simulink model "stand_nove"  (R2021a)
settings: Solver=VariableStepAuto  StartTime=0.0  StopTime=3.0  RelTol=1e-3
values from neighbouring files (symbols this model uses):
  fn = 50    [stand_final.m]
  Jm = 0.0019    [stand_final.m]
  pp = 2    [stand_final.m]
  Un = 23.4    [stand_final.m]
  X0 = 0    [stand_final.m]
libraries: General x38, nesl_utility x16, Math x12, ee_lib x11, fl_lib x11, Control x4, MotorControl x3, Basic x1
settings Model: Creator=pavel  LastModifiedBy=pavel

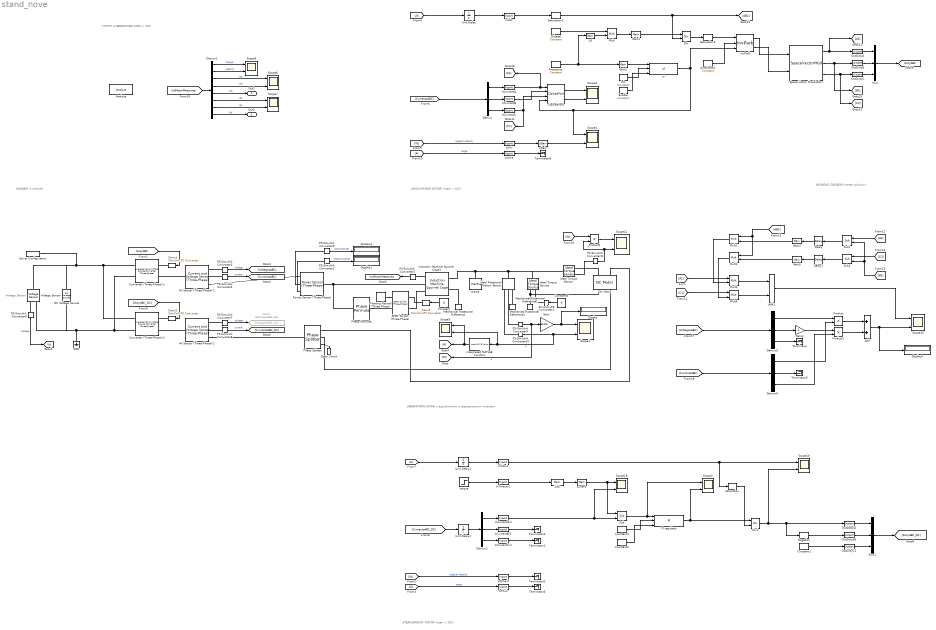
== system stand_nove ==
  note: ASYNCHRONNI MOTOR
      | (rizeni v X2C)
  note: LABORATORNI STAND
      | s asynchronnim a stejnosmernym motorem
  note: Voltage Sensor
  note: STEJNOSMERNY MOTOR
      | (rizeni v X2C)
  note: NAPAJENI
      | (z menice)
  note: ARONOVO ZAPOJENI
      | (mereni prikonu)
  note: VYSTUP a GENEROVANI KODU v X2C
  1/cfi : General/Gain  Gain=1/0.06  M2CAutoParam_UsedImplementation=32 Bit Floating Point  x2c_cfg_enableStaticId=off  x2c_cfg_staticId=1  x2c_cfg_enableCot=off  BlockName=Gain
      settings: SourceProductName=X2C General
  1/f : General/Gain  Gain=1/fn  M2CAutoParam_UsedImplementation=32 Bit Floating Point  x2c_cfg_enableStaticId=off  x2c_cfg_staticId=1  x2c_cfg_enableCot=off  BlockName=Gain
      settings: SourceProductName=X2C General
  AV Sensor (Three-Phase)-1 : ee_lib/Sensors & Transducers/Current and Voltage Sensor (Three-Phase)  vMeasurementType=ee.enum.vmeasurement.ll  outputUnit=ee.enum.unit.si  SRated=100e6 V*A  VRated=24e3 V  I_specify=off  I_priority=None  I=[ 0 0 0 ] A  I_nominal_specify=off  I_nominal_unit=A  I_nominal_value=1  V_specify=off  V_priority=None  V=[ 0 0 0 ] V  V_nominal_specify=off  V_nominal_unit=V  V_nominal_value=1
      settings: SourceProductBaseCode=PS  InternalSimscapePortConfiguration="{\"Bottom\":[],\"Left\":[{\"id\":\"N1\",\"label\":\"~1\",\"type\":\"foundation.electrical.three_phase\"}],\"Right\":[{\"id\":\"V_output\",\"label\":\"V\",\"type\":\"output\"},{\"id\":\"I_output\",\"label\":\"I\",\"type\":\"output\"},{\"id\":\"N2\",\"label\":\"~2\",\"type\":\"foundation.electrical.three_phase\"}],\"Top\":[]}"
  AV Sensor (Three-Phase)-2 : ee_lib/Sensors & Transducers/Current and Voltage Sensor (Three-Phase)  vMeasurementType=ee.enum.vmeasurement.ll  outputUnit=ee.enum.unit.si  SRated=100e6 V*A  VRated=24e3 V  I_specify=off  I_priority=None  I=[ 0 0 0 ] A  I_nominal_specify=off  I_nominal_unit=A  I_nominal_value=1  V_specify=off  V_priority=None  V=[ 0 0 0 ] V  V_nominal_specify=off  V_nominal_unit=V  V_nominal_value=1
      settings: SourceProductBaseCode=PS  InternalSimscapePortConfiguration="{\"Bottom\":[],\"Left\":[{\"id\":\"N1\",\"label\":\"~1\",\"type\":\"foundation.electrical.three_phase\"}],\"Right\":[{\"id\":\"V_output\",\"label\":\"V\",\"type\":\"output\"},{\"id\":\"I_output\",\"label\":\"I\",\"type\":\"output\"},{\"id\":\"N2\",\"label\":\"~2\",\"type\":\"foundation.electrical.three_phase\"}],\"Top\":[]}"
  Add : Sum
  Add1 : Math/Add  M2CAutoParam_UsedImplementation=32 Bit Floating Point  x2c_cfg_enableStaticId=off  x2c_cfg_staticId=1  x2c_cfg_enableCot=off  BlockName=Add
      settings: SourceProductName=X2C Math
  Amplitude1 : General/Constant  Value=0  M2CAutoParam_UsedImplementation=32 Bit Floating Point  x2c_cfg_enableStaticId=off  x2c_cfg_staticId=1  x2c_cfg_enableCot=off  BlockName=Constant
      settings: SourceProductName=X2C General
  Analyze : Basic/Analyze
      settings: SourceProductName=X2C Basic
  ClarkeNPark : MotorControl/ClarkeNPark  M2CAutoParam_UsedImplementation=32 Bit Floating Point  x2c_cfg_enableStaticId=off  x2c_cfg_staticId=1  x2c_cfg_enableCot=off  BlockName=ClarkeNPark
      settings: SourceProductName=X2C MotorControl
  Constant : Constant  Value=0
  Constant1 : General/Constant  Value=0.0  M2CAutoParam_UsedImplementation=32 Bit Floating Point  x2c_cfg_enableStaticId=off  x2c_cfg_staticId=1  x2c_cfg_enableCot=off  BlockName=Constant
      settings: SourceProductName=X2C General
  Constant3 : General/Constant  Value=1  M2CAutoParam_UsedImplementation=Boolean  x2c_cfg_enableStaticId=off  x2c_cfg_staticId=1  x2c_cfg_enableCot=off  BlockName=Constant
      settings: SourceProductName=X2C General
  Constant4 : General/Constant  Value=0.0  M2CAutoParam_UsedImplementation=32 Bit Floating Point  x2c_cfg_enableStaticId=off  x2c_cfg_staticId=1  x2c_cfg_enableCot=off  BlockName=Constant
      settings: SourceProductName=X2C General
  Constant6 : Constant  Value=0
  Conv1 : nesl_utility/Simulink-PS Converter  PhysicalDomain=network_engine_domain  SubClassName=ps_input  LeftPortType=input  RightPortType=output  PseudoPeriodic=off  Frequencies=[]  NoiseDistribution=none  NoiseParameters=[]  Unit=1  AffineConversion=off  FilteringAndDerivatives=provide  SimscapeFilterOrder=1  InputFilterTimeConstant=0.001  UdotUserProvided=0
      settings: SourceProductBaseCode=PW,SS
  Conv2 : nesl_utility/Simulink-PS Converter  PhysicalDomain=network_engine_domain  SubClassName=ps_input  LeftPortType=input  RightPortType=output  PseudoPeriodic=off  Frequencies=[]  NoiseDistribution=none  NoiseParameters=[]  Unit=1  AffineConversion=off  FilteringAndDerivatives=provide  SimscapeFilterOrder=1  InputFilterTimeConstant=0.001  UdotUserProvided=0
      settings: SourceProductBaseCode=PW,SS
  Conv3 : nesl_utility/Simulink-PS Converter  PhysicalDomain=network_engine_domain  SubClassName=ps_input  LeftPortType=input  RightPortType=output  PseudoPeriodic=off  Frequencies=[]  NoiseDistribution=none  NoiseParameters=[]  Unit=1  AffineConversion=off  FilteringAndDerivatives=provide  SimscapeFilterOrder=1  InputFilterTimeConstant=0.001  UdotUserProvided=0
      settings: SourceProductBaseCode=PW,SS
  Converter (Three-Phase)-1 : ee_lib/Semiconductors & Converters/Converters/Average-Value Voltage Source Converter (Three-Phase)  losses_parameterization=ee.enum.converters.losses.fixed  Pfixed=0.0001 W  ks=0.01  kc1=1.7 V  kc2=0.01 Ohm  Ploss_vect=[100, 800, 1870, 3250, 4900] W  Irms_vect=[10, 100, 200, 300, 400] A  Vdc_nom=300 V  thermal_mass=30000 J/K  temperature_specify=off  temperature_priority=High  temperature=298.15 K  temperature_nominal_specify=off  temperature_nominal_unit=K  temperature_nominal_value=1
      settings: SourceProductBaseCode=PS  InternalSimscapePortConfiguration="{\"Bottom\":[],\"Left\":[{\"id\":\"ModWave\",\"label\":\"ModWave\",\"type\":\"input\"},{\"id\":\"N\",\"label\":\"~\",\"type\":\"foundation.electrical.three_phase\"}],\"Right\":[{\"id\":\"p\",\"label\":\"+\",\"type\":\"foundation.electrical.electrical\"},{\"id\":\"n\",\"label\":\"-\",\"type\":\"foundation.electrical.electrical\"}],\"Top\":[]}"
  Converter (Three-Phase)-2 : ee_lib/Semiconductors & Converters/Converters/Average-Value Voltage Source Converter (Three-Phase)  losses_parameterization=ee.enum.converters.losses.fixed  Pfixed=0.1 W  ks=0.01  kc1=1.7 V  kc2=0.01 Ohm  Ploss_vect=[100, 800, 1870, 3250, 4900] W  Irms_vect=[10, 100, 200, 300, 400] A  Vdc_nom=300 V  thermal_mass=30000 J/K  temperature_specify=off  temperature_priority=High  temperature=298.15 K  temperature_nominal_specify=off  temperature_nominal_unit=K  temperature_nominal_value=1
      settings: SourceProductBaseCode=PS  InternalSimscapePortConfiguration="{\"Bottom\":[],\"Left\":[{\"id\":\"ModWave\",\"label\":\"ModWave\",\"type\":\"input\"},{\"id\":\"N\",\"label\":\"~\",\"type\":\"foundation.electrical.three_phase\"}],\"Right\":[{\"id\":\"p\",\"label\":\"+\",\"type\":\"foundation.electrical.electrical\"},{\"id\":\"n\",\"label\":\"-\",\"type\":\"foundation.electrical.electrical\"}],\"Top\":[]}"
  DC Voltage Source : fl_lib/Electrical/Electrical Sources/DC Voltage Source  v0=Ud V
  DC Motor : ee_lib/Electromechanical/Brushed Motors/DC Motor  field_option=ee.enum.field_option.pm  Rf=100 Ohm  Lf=1 H  Laf=0.15 H  If0=0 A  parameterization=ee.enum.dcparam_option.circuit_param  Ra=Ra Ohm  La=La H  emf_or_torque=ee.enum.emf_or_torque.kv  Kv=cfi V/(rad/s)  Ki=6.876e-4 N*m/A  T_stall=0.24e-3 N*m  w_max=19100 rpm  w_rated=15000 rpm  P_rated=0.08 W  V_rated=1.5 V  J=Jm kg*m^2  lam_param=ee.enum.lam_param.damping  lam=0 N*m/(rad/s)  i_noload=0 A  V_i_noload=1.5 V  speed0=0 rpm  enable_fault_armature=ee.enum.faults.faultEnable.no  rev_faulted=1 / 3  G_faulted_armature=1e-5 S  fault_trigger_armature=ee.enum.faults.faultTrigger.temporal  t_fault_armature=1 s  max_permissible_current_armature=inf A  t_fail_on_current_armature=1 s  enable_fault_field=ee.enum.faults.faultEnable.no  G_faulted_field=1e-5 S  fault_trigger_field=ee.enum.faults.faultTrigger.temporal  t_fault_field=1 s  max_permissible_current_field=inf A  t_fail_on_current_field=1 s  fault_action=ee.enum.faults.faultAction.none  alpha=3.93e-3 1/K  Tmeas=25 degC  thermal_mass=100 J/K  initial_temperature=25 degC
  Delay : Control/Delay  ts_fact=1.0  M2CAutoParam_UsedImplementation=32 Bit Floating Point  x2c_cfg_enableStaticId=off  x2c_cfg_staticId=1  x2c_cfg_enableCot=off  BlockName=Delay
      settings: SourceProductName=X2C Control
  Delay1 : Control/Delay  ts_fact=1.0  M2CAutoParam_UsedImplementation=32 Bit Floating Point  x2c_cfg_enableStaticId=off  x2c_cfg_staticId=1  x2c_cfg_enableCot=off  BlockName=Delay
      settings: SourceProductName=X2C Control
  Demux{,2,5..6} (4 alike) : Demux  Outputs=3
  Demux1 : Demux  Outputs=8
  Display{,1,3..4} (4 alike) : Display
  Div : Math/Div  M2CAutoParam_UsedImplementation=32 Bit Floating Point  x2c_cfg_enableStaticId=off  x2c_cfg_staticId=1  x2c_cfg_enableCot=off  BlockName=Div
      settings: SourceProductName=X2C Math
  Div1 : Math/Div  M2CAutoParam_UsedImplementation=32 Bit Floating Point  x2c_cfg_enableStaticId=off  x2c_cfg_staticId=1  x2c_cfg_enableCot=off  BlockName=Div
      settings: SourceProductName=X2C Math
  Enable : General/Constant  Value=1  M2CAutoParam_UsedImplementation=Boolean  x2c_cfg_enableStaticId=off  x2c_cfg_staticId=1  x2c_cfg_enableCot=off  BlockName=Constant
      settings: SourceProductName=X2C General
  Floating Neutral (Three-Phase) : ee_lib/Connectors & References/Floating Neutral (Three-Phase)  G_parasitic=1e-12 1/Ohm
      settings: SourceProductBaseCode=PS  InternalSimscapePortConfiguration="{\"Bottom\":[],\"Left\":[{\"id\":\"N\",\"label\":\"~\",\"type\":\"foundation.electrical.three_phase\"}],\"Right\":[],\"Top\":[]}"
  Frequency : General/Constant  Value=fn  M2CAutoParam_UsedImplementation=32 Bit Floating Point  x2c_cfg_enableStaticId=off  x2c_cfg_staticId=1  x2c_cfg_enableCot=off  BlockName=Constant
      settings: SourceProductName=X2C General
  GND : fl_lib/Electrical/Electrical Elements/Electrical Reference
  Gain : Gain  Gain=60/2/pi
  Gain1 : General/Gain  Gain=1.44  M2CAutoParam_UsedImplementation=32 Bit Floating Point  x2c_cfg_enableStaticId=off  x2c_cfg_staticId=1  x2c_cfg_enableCot=off  BlockName=Gain
      settings: SourceProductName=X2C General
  Gain2 : General/Gain  Gain=2*pi  M2CAutoParam_UsedImplementation=32 Bit Floating Point  x2c_cfg_enableStaticId=off  x2c_cfg_staticId=1  x2c_cfg_enableCot=off  BlockName=Gain
      settings: SourceProductName=X2C General
  Gain3 : Gain  Gain=-1
  Gain4 : General/Gain  Gain=0.5  M2CAutoParam_UsedImplementation=32 Bit Floating Point  x2c_cfg_enableStaticId=off  x2c_cfg_staticId=1  x2c_cfg_enableCot=off  BlockName=Gain
      settings: SourceProductName=X2C General
  Gain5 : General/Gain  Gain=0.5  M2CAutoParam_UsedImplementation=32 Bit Floating Point  x2c_cfg_enableStaticId=off  x2c_cfg_staticId=1  x2c_cfg_enableCot=off  BlockName=Gain
      settings: SourceProductName=X2C General
  Goto2 : Goto  Commented=on  GotoTag=VoltagesABC_DC
  Ideal Rotational Motion Sensor : fl_lib/Mechanical/Mechanical Sensors/Ideal Rotational Motion Sensor  wrap_angle=simscape.enum.onoff.off  offset=0 rad
  Ideal Torque Sensor : fl_lib/Mechanical/Mechanical Sensors/Ideal Torque Sensor
  Ideal Torque Source : fl_lib/Mechanical/Mechanical Sources/Ideal Torque Source
  InCurrentA : General/Inport  DataType=float32  ts_fact=1.0  x2c_cfg_enableStaticId=off  x2c_cfg_staticId=0  BlockName=Inport  gain=1  offset=0
      settings: SourceProductName=X2C General
  InCurrentA-2 : General/Inport  DataType=float32  ts_fact=1.0  x2c_cfg_enableStaticId=off  x2c_cfg_staticId=0  BlockName=Inport  gain=1  offset=0
      settings: SourceProductName=X2C General
  InCurrentB : General/Inport  DataType=float32  ts_fact=1.0  x2c_cfg_enableStaticId=off  x2c_cfg_staticId=0  BlockName=Inport  gain=1  offset=0
      settings: SourceProductName=X2C General
  InCurrentB-2 : General/Inport  DataType=float32  ts_fact=1.0  x2c_cfg_enableStaticId=off  x2c_cfg_staticId=0  BlockName=Inport  gain=1  offset=0
      settings: SourceProductName=X2C General
  InCurrentC : General/Inport  DataType=float32  ts_fact=1.0  x2c_cfg_enableStaticId=off  x2c_cfg_staticId=0  BlockName=Inport  gain=1  offset=0
      settings: SourceProductName=X2C General
  InCurrentC-2 : General/Inport  DataType=float32  ts_fact=1.0  x2c_cfg_enableStaticId=off  x2c_cfg_staticId=0  BlockName=Inport  gain=1  offset=0
      settings: SourceProductName=X2C General
  InOme : General/Inport  DataType=float32  ts_fact=1.0  x2c_cfg_enableStaticId=off  x2c_cfg_staticId=0  BlockName=Inport  gain=1  offset=0
      settings: SourceProductName=X2C General
  InOme-2 : General/Inport  DataType=float32  ts_fact=1.0  x2c_cfg_enableStaticId=off  x2c_cfg_staticId=0  BlockName=Inport  gain=1  offset=0
      settings: SourceProductName=X2C General
  InPhi : General/Inport  DataType=float32  ts_fact=1.0  x2c_cfg_enableStaticId=off  x2c_cfg_staticId=0  BlockName=Inport  gain=1  offset=0
      settings: SourceProductName=X2C General
  InPhi-2 : General/Inport  DataType=float32  ts_fact=1.0  x2c_cfg_enableStaticId=off  x2c_cfg_staticId=0  BlockName=Inport  gain=1  offset=0
      settings: SourceProductName=X2C General
  InTorque-2 : General/Inport  DataType=float32  ts_fact=1.0  x2c_cfg_enableStaticId=off  x2c_cfg_staticId=0  BlockName=Inport  gain=1  offset=0
      settings: SourceProductName=X2C General
  InVdc : General/Inport  DataType=float32  ts_fact=1.0  x2c_cfg_enableStaticId=off  x2c_cfg_staticId=0  BlockName=Inport  gain=1  offset=0
      settings: SourceProductName=X2C General
  InVdc-2 : General/Inport  DataType=float32  ts_fact=1.0  x2c_cfg_enableStaticId=off  x2c_cfg_staticId=0  BlockName=Inport  gain=1  offset=0
      settings: SourceProductName=X2C General
  Induction Machine Squirrel Cage1 : ee_lib/Electromechanical/Asynchronous/Induction Machine Squirrel Cage  SRated=Pn W  VRated=Un V  FRated=fn Hz  nPolePairs=pp  param_unit=ee.enum.unit.si  squirrel_cage=ee.enum.squirrelcage.Single  zero_sequence=ee.enum.park.zerosequence.include  Rs=Rs Ohm  Xls=Xls Ohm  pu_Rs=0.0258  pu_Lls=0.0413  Rrd=Rr Ohm  Xlrd=Xlr Ohm  pu_Rrd=0.0145  pu_Llrd=0.0424  Rrd1=0.28 Ohm  Xlrd1=0.82 Ohm  Rrd2=0.28 Ohm  Xlrd2=0.82 Ohm  pu_Rrd1=0.0290  pu_Llrd1=0.0848  pu_Rrd2=0.0290  pu_Llrd2=0.0848  Xm=Xm Ohm  pu_Lm=1.7562  X0=X0 Ohm  pu_L0=0.0413  saturation_option=ee.enum.saturation.exclude  saturation_i=[0, 4, 9, 18, 25, 34, 50, 68, 95, 120] A  saturation_v=[0, 88, 154, 198, 220, 242, 264, 286, 308, 327] V  pu_saturation_i=[0, .176, .396, .792, 1.1, 1.496, 2.2, 2.992, 4.18, 5.28]  pu_saturation_v=[0, .4, .7, .9, 1, 1.1, 1.2, 1.3, 1.4, 1.4864]  initialization_option=ee.enum.asm.initialization.fluxvariables  connection_option=ee.enum.Connection.delta  angular_position_specify=off  angular_position_priority=None  angular_position=0 deg  angular_position_nominal_specify=off  angular_position_nominal_unit=deg  angular_position_nominal_value=1  pu_psids_specify=off  pu_psids_priority=None  pu_psids=0  pu_psids_nominal_specify=off  pu_psids_nominal_unit=1  pu_psids_nominal_value=1  pu_psiqs_specify=off  pu_psiqs_priority=None  pu_psiqs=0  pu_psiqs_nominal_specify=off  pu_psiqs_nominal_unit=1  pu_psiqs_nominal_value=1  pu_psi0s_specify=off  pu_psi0s_priority=None  pu_psi0s=0  pu_psi0s_nominal_specify=off  pu_psi0s_nominal_unit=1  pu_psi0s_nominal_value=1  pu_psidr_specify=off  pu_psidr_priority=None  pu_psidr=0  pu_psidr_nominal_specify=off  pu_psidr_nominal_unit=1  pu_psidr_nominal_value=1  pu_psiqr_specify=off  pu_psiqr_priority=None  pu_psiqr=0  pu_psiqr_nominal_specify=off  pu_psiqr_nominal_unit=1  pu_psiqr_nominal_value=1  pu_psidr1_specify=off  pu_psidr1_priority=None  pu_psidr1=0  pu_psidr1_nominal_specify=off  pu_psidr1_nominal_unit=1  pu_psidr1_nominal_value=1  pu_psiqr1_specify=off  pu_psiqr1_priority=None  pu_psiqr1=0  pu_psiqr1_nominal_specify=off  pu_psiqr1_nominal_unit=1  pu_psiqr1_nominal_value=1  pu_psidr2_specify=off  pu_psidr2_priority=None  pu_psidr2=0  pu_psidr2_nominal_specify=off  pu_psidr2_nominal_unit=1  pu_psidr2_nominal_value=1  pu_psiqr2_specify=off  pu_psiqr2_priority=None  pu_psiqr2=0  pu_psiqr2_nominal_specify=off  pu_psiqr2_nominal_unit=1  pu_psiqr2_nominal_value=1  psids_specify=off  psids_priority=None  psids=0 Wb  psids_nominal_specify=off  psids_nominal_unit=Wb  psids_nominal_value=1  psiqs_specify=off  psiqs_priority=None  psiqs=0 Wb  psiqs_nominal_specify=off  psiqs_nominal_unit=Wb  psiqs_nominal_value=1  psi0s_specify=off  psi0s_priority=None  psi0s=0 Wb  psi0s_nominal_specify=off  psi0s_nominal_unit=Wb  psi0s_nominal_value=1  psidr_specify=off  psidr_priority=None  psidr=0 Wb  psidr_nominal_specify=off  psidr_nominal_unit=Wb  psidr_nominal_value=1  psiqr_specify=off  psiqr_priority=None  psiqr=0 Wb  psiqr_nominal_specify=off  psiqr_nominal_unit=Wb  psiqr_nominal_value=1  psidr1_specify=off  psidr1_priority=None  psidr1=0 Wb  psidr1_nominal_specify=off  psidr1_nominal_unit=Wb  psidr1_nominal_value=1  psiqr1_specify=off  psiqr1_priority=None  psiqr1=0 Wb  psiqr1_nominal_specify=off  psiqr1_nominal_unit=Wb  psiqr1_nominal_value=1  psidr2_specify=off  psidr2_priority=None  psidr2=0 Wb  psidr2_nominal_specify=off  psidr2_nominal_unit=Wb  psidr2_nominal_value=1  psiqr2_specify=off  psiqr2_priority=None  psiqr2=0 Wb  psiqr2_nominal_specify=off  psiqr2_nominal_unit=Wb  psiqr2_nominal_value=1  slip_specify=off  slip_priority=None  slip=0  slip_nominal_specify=off  slip_nominal_unit=1  slip_nominal_value=1  real_power_generated_specify=off  real_power_generated_priority=None  real_power_generated=0 W  real_power_generated_nominal_specify=off  real_power_generated_nominal_unit=W  real_power_generated_nominal_value=1  mechanical_power_consumed_specify=off  mechanical_power_consumed_priority=None  mechanical_power_consumed=0 W  mechanical_power_consumed_nominal_specify=off  mechanical_power_consumed_nominal_unit=W  mechanical_power_consumed_nominal_value=1
      settings: SourceProductBaseCode=PS  InternalSimscapePortConfiguration="{\"Bottom\":[],\"Left\":[{\"id\":\"R\",\"label\":\"R\",\"type\":\"foundation.mechanical.rotational.rotational\"},{\"id\":\"C\",\"label\":\"C\",\"type\":\"foundation.mechanical.rotational.rotational\"}],\"Right\":[{\"id\":\"pu_output\",\"label\":\"pu\",\"type\":\"output\"},{\"id\":\"N1\",\"label\":\"~1\",\"type\":\"foundation.electrical.three_phase\"},{\"id\":\"N2\",\"label\":\"~2\",\"type\":\"foundation.electrical.three_phase\"}],\"Top\":[]}"
  Inertia : fl_lib/Mechanical/Rotational Elements/Inertia  inertia=0.0004 kg*m^2  num_ports=foundation.enum.numPorts2.one  w_specify=off  w_priority=High  w=0 rad/s  w_nominal_specify=off  w_nominal_unit=rad/s  w_nominal_value=1  t_specify=off  t_priority=None  t=0 N*m  t_nominal_specify=off  t_nominal_unit=N*m  t_nominal_value=1
  Init : General/Constant  Value=0  M2CAutoParam_UsedImplementation=32 Bit Floating Point  x2c_cfg_enableStaticId=off  x2c_cfg_staticId=1  x2c_cfg_enableCot=off  BlockName=Constant
      settings: SourceProductName=X2C General
  Interpreted MATLAB Function : MATLABFcn  MATLABFcn=mod(u(1),2*pi)-pi
  InvPark : MotorControl/InvPark  M2CAutoParam_UsedImplementation=32 Bit Floating Point  x2c_cfg_enableStaticId=off  x2c_cfg_staticId=1  x2c_cfg_enableCot=off  BlockName=InvPark
      settings: SourceProductName=X2C MotorControl
  Mechanical Rotational Reference : fl_lib/Mechanical/Rotational Elements/Mechanical Rotational Reference
  Mechanical Rotational Reference1 : fl_lib/Mechanical/Rotational Elements/Mechanical Rotational Reference
  Mechanical Rotational Reference2 : fl_lib/Mechanical/Rotational Elements/Mechanical Rotational Reference
  Mult{,1..3,5} (5 alike) : Math/Mult  M2CAutoParam_UsedImplementation=32 Bit Floating Point  x2c_cfg_enableStaticId=off  x2c_cfg_staticId=1  x2c_cfg_enableCot=off  BlockName=Mult
      settings: SourceProductName=X2C Math
  Mux : Mux  Inputs=3
  Mux1 : Mux  Inputs=3
  Negation : Math/Negation  M2CAutoParam_UsedImplementation=32 Bit Floating Point  x2c_cfg_enableStaticId=off  x2c_cfg_staticId=1  x2c_cfg_enableCot=off  BlockName=Negation
      settings: SourceProductName=X2C Math
  Open Circuit : fl_lib/Electrical/Electrical Elements/Open Circuit  v_specify=off  v_priority=None  v=0 V  v_nominal_specify=off  v_nominal_unit=V  v_nominal_value=1
      settings: SourceProductBaseCode=SS
  OutDutyA : General/Outport  DataType=float32  ts_fact=1.0  x2c_cfg_enableStaticId=off  x2c_cfg_staticId=0  BlockName=Outport  gain=1  offset=0
      settings: SourceProductName=X2C General
  OutDutyA1 : General/Outport  DataType=float32  ts_fact=1.0  x2c_cfg_enableStaticId=off  x2c_cfg_staticId=0  BlockName=Outport  gain=1  offset=0
      settings: SourceProductName=X2C General
  OutDutyB : General/Outport  DataType=float32  ts_fact=1.0  x2c_cfg_enableStaticId=off  x2c_cfg_staticId=0  BlockName=Outport  gain=1  offset=0
      settings: SourceProductName=X2C General
  OutDutyB1 : General/Outport  DataType=float32  ts_fact=1.0  x2c_cfg_enableStaticId=off  x2c_cfg_staticId=0  BlockName=Outport  gain=1  offset=0
      settings: SourceProductName=X2C General
  OutDutyC : General/Outport  DataType=float32  ts_fact=1.0  x2c_cfg_enableStaticId=off  x2c_cfg_staticId=0  BlockName=Outport  gain=1  offset=0
      settings: SourceProductName=X2C General
  OutDutyC1 : General/Outport  DataType=float32  ts_fact=1.0  x2c_cfg_enableStaticId=off  x2c_cfg_staticId=0  BlockName=Outport  gain=1  offset=0
      settings: SourceProductName=X2C General
  PI regulátor : Control/PI  Kp=1.67  Ki=733  ts_fact=1.0  M2CAutoParam_UsedImplementation=32 Bit Floating Point  x2c_cfg_enableStaticId=off  x2c_cfg_staticId=1  x2c_cfg_enableCot=off  BlockName=PI
      settings: SourceProductName=X2C Control
  PS-Simulink Converter{1..11} (11 alike) : nesl_utility/PS-Simulink Converter  PhysicalDomain=network_engine_domain  SubClassName=ps_output  LeftPortType=input  RightPortType=output  PseudoPeriodic=off  Frequencies=[]  Unit=inherit  AffineConversion=off
      settings: SourceProductBaseCode=PW,SS
  Phase Permute : ee_lib/Connectors & References/Phase Permute
      settings: SourceProductBaseCode=PS  InternalSimscapePortConfiguration="{\"Bottom\":[],\"Left\":[{\"id\":\"N123\",\"label\":\"~123\",\"type\":\"foundation.electrical.three_phase\"}],\"Right\":[{\"id\":\"N231\",\"label\":\"~231\",\"type\":\"foundation.electrical.three_phase\"}],\"Top\":[]}"
  Phase Splitter : ee_lib/Connectors & References/Phase Splitter
      settings: SourceProductBaseCode=PS
  Power Sensor (Three-Phase) : ee_lib/Sensors & Transducers/Power Sensor (Three-Phase)  load_type=ee.enum.passive.type_balanced.balanced  f0=50 Hz  config=ee.enum.with_neutral.no  rho=1
      settings: SourceProductBaseCode=PS  InternalSimscapePortConfiguration="{\"Bottom\":[],\"Left\":[{\"id\":\"N1\",\"label\":\"~1\",\"type\":\"foundation.electrical.three_phase\"}],\"Right\":[{\"id\":\"N2\",\"label\":\"~2\",\"type\":\"foundation.electrical.three_phase\"}],\"Top\":[{\"id\":\"Pm\",\"label\":\"P\",\"type\":\"output\"},{\"id\":\"Qm\",\"label\":\"Q\",\"type\":\"output\"}]}"
  Product : Product
  Product1 : Product
  Product2 : Product
  SPDT Switch (Three-Phase) : ee_lib/Switches & Breakers/SPDT Switch (Three-Phase)  R_closed=0.001 Ohm  G_open=1e-6 1/Ohm  threshold=0.5 V  i_vT_specify=off  i_vT_priority=None  i_vT=0 A  i_vT_nominal_specify=off  i_vT_nominal_unit=A  i_vT_nominal_value=1  I12_specify=off  I12_priority=None  I12=[0, 0, 0] A  I12_nominal_specify=off  I12_nominal_unit=A  I12_nominal_value=1  V12_specify=off  V12_priority=None  V12=[0, 0, 0] V  V12_nominal_specify=off  V12_nominal_unit=V  V12_nominal_value=1  I13_specify=off  I13_priority=None  I13=[0, 0, 0] A  I13_nominal_specify=off  I13_nominal_unit=A  I13_nominal_value=1  V13_specify=off  V13_priority=None  V13=[0, 0, 0] V  V13_nominal_specify=off  V13_nominal_unit=V  V13_nominal_value=1  i_a_12_specify=off  i_a_12_priority=None  i_a_12=0 A  i_a_12_nominal_specify=off  i_a_12_nominal_unit=A  i_a_12_nominal_value=1  v_a_12_specify=off  v_a_12_priority=None  v_a_12=0 V  v_a_12_nominal_specify=off  v_a_12_nominal_unit=V  v_a_12_nominal_value=1  i_a_13_specify=off  i_a_13_priority=None  i_a_13=0 A  i_a_13_nominal_specify=off  i_a_13_nominal_unit=A  i_a_13_nominal_value=1  v_a_13_specify=off  v_a_13_priority=None  v_a_13=0 V  v_a_13_nominal_specify=off  v_a_13_nominal_unit=V  v_a_13_nominal_value=1  i_b_12_specify=off  i_b_12_priority=None  i_b_12=0 A  i_b_12_nominal_specify=off  i_b_12_nominal_unit=A  i_b_12_nominal_value=1  v_b_12_specify=off  v_b_12_priority=None  v_b_12=0 V  v_b_12_nominal_specify=off  v_b_12_nominal_unit=V  v_b_12_nominal_value=1  i_b_13_specify=off  i_b_13_priority=None  i_b_13=0 A  i_b_13_nominal_specify=off  i_b_13_nominal_unit=A  i_b_13_nominal_value=1  v_b_13_specify=off  v_b_13_priority=None  v_b_13=0 V  v_b_13_nominal_specify=off  v_b_13_nominal_unit=V  v_b_13_nominal_value=1  i_c_12_specify=off  i_c_12_priority=None  i_c_12=0 A  i_c_12_nominal_specify=off  i_c_12_nominal_unit=A  i_c_12_nominal_value=1  v_c_12_specify=off  v_c_12_priority=None  v_c_12=0 V  v_c_12_nominal_specify=off  v_c_12_nominal_unit=V  v_c_12_nominal_value=1  i_c_13_specify=off  i_c_13_priority=None  i_c_13=0 A  i_c_13_nominal_specify=off  i_c_13_nominal_unit=A  i_c_13_nominal_value=1  v_c_13_specify=off  v_c_13_priority=None  v_c_13=0 V  v_c_13_nominal_specify=off  v_c_13_nominal_unit=V  v_c_13_nominal_value=1
      settings: SourceProductBaseCode=PS  InternalSimscapePortConfiguration="{\"Bottom\":[],\"Left\":[{\"id\":\"vT\",\"label\":\"vT\",\"type\":\"input\"},{\"id\":\"N1\",\"label\":\"~1\",\"type\":\"foundation.electrical.three_phase\"}],\"Right\":[{\"id\":\"N2\",\"label\":\"~2\",\"type\":\"foundation.electrical.three_phase\"},{\"id\":\"N3\",\"label\":\"~3\",\"type\":\"foundation.electrical.three_phase\"}],\"Top\":[]}"
  Saturation : General/Saturation  max=35  min=10  M2CAutoParam_UsedImplementation=32 Bit Floating Point  x2c_cfg_enableStaticId=off  x2c_cfg_staticId=1  x2c_cfg_enableCot=off  BlockName=Saturation
      settings: SourceProductName=X2C General
  Saturation1 : General/Saturation  max=60  min=10  M2CAutoParam_UsedImplementation=32 Bit Floating Point  x2c_cfg_enableStaticId=off  x2c_cfg_staticId=1  x2c_cfg_enableCot=off  BlockName=Saturation
      settings: SourceProductName=X2C General
  Saturation2 : General/Saturation  max=1  min=-1  M2CAutoParam_UsedImplementation=32 Bit Floating Point  x2c_cfg_enableStaticId=off  x2c_cfg_staticId=1  x2c_cfg_enableCot=off  BlockName=Saturation
      settings: SourceProductName=X2C General
  Scope{1..7,9..10,12,15,18} (12 alike) : Scope  NumInputPorts=2
  Simulink-PS Converter1 : nesl_utility/Simulink-PS Converter  PhysicalDomain=network_engine_domain  SubClassName=ps_input  LeftPortType=input  RightPortType=output  PseudoPeriodic=off  Frequencies=[]  NoiseDistribution=none  NoiseParameters=[]  Unit=1  AffineConversion=off  FilteringAndDerivatives=provide  SimscapeFilterOrder=1  InputFilterTimeConstant=0.001  UdotUserProvided=0
      settings: SourceProductBaseCode=PW,SS
  Solver Configuration : nesl_utility/Solver Configuration  PhysicalDomain=network_engine_domain  SubClassName=solver  LeftPortType=input  RightPortType=generic  Tones=[]  Harmonics=[]  SimulateNoise=off  Profile=off  UseLocalSampling=off  EnableSwitchedLinearOptims=on  FrequencyDomain=off  UseCCode=off  RelTol=0.001  AbsTol=1e-06  MinStep=1e-09  ToWorkspace=off  RevertToSquareIcSolve=off  NumHomotopyIterations=100  PhasorMode=off  PhasorModeNumHarmonics=1  DoDC=off  ResidualTolerance=1e-09  UseLocalSolver=on  LocalSolverChoice=NE_BACKWARD_EULER_ADVANCER  LocalSolverSampleTime=0.00005  DoFixedCost=on  MaxNonlinIter=3  MaxModeIter=2  ComputeImpulses=off  ImpulseIterations=2  LinearAlgebra=auto  EquationFormulation=NE_TIME_EF  DelaysMemoryBudget=1024  AutomaticFiltering=on  FilteringTimeConstant=0.001  PartitionStorageMethod=AS_NEEDED  PartitionMemoryBudget=1024  PartitionMethod=ROBUST
      settings: SourceProductBaseCode=PW,SS
  Space Vector Modulation : MotorControl/SpaceVectorMod  method=Alternating reversing  M2CAutoParam_UsedImplementation=32 Bit Floating Point  x2c_cfg_enableStaticId=off  x2c_cfg_staticId=1  x2c_cfg_enableCot=off  BlockName=SpaceVectorMod
      settings: SourceProductName=X2C MotorControl
  Sub : Math/Sub  M2CAutoParam_UsedImplementation=32 Bit Floating Point  x2c_cfg_enableStaticId=off  x2c_cfg_staticId=1  x2c_cfg_enableCot=off  BlockName=Sub
      settings: SourceProductName=X2C Math
  Sub1 : Math/Sub  M2CAutoParam_UsedImplementation=32 Bit Floating Point  x2c_cfg_enableStaticId=off  x2c_cfg_staticId=1  x2c_cfg_enableCot=off  BlockName=Sub
      settings: SourceProductName=X2C Math
  Sub2 : Math/Sub  M2CAutoParam_UsedImplementation=32 Bit Floating Point  x2c_cfg_enableStaticId=off  x2c_cfg_staticId=1  x2c_cfg_enableCot=off  BlockName=Sub
      settings: SourceProductName=X2C Math
  Terminator{,1..5,8} (7 alike) : Terminator
  Unit Delay : UnitDelay  SampleTime=-1  HasFrameUpgradeWarning=on
  Unit Delay1 : UnitDelay  SampleTime=-1  HasFrameUpgradeWarning=on
  Unit Delay2 : UnitDelay  SampleTime=-1  HasFrameUpgradeWarning=on
  Voltage : General/Constant  Value=Un  M2CAutoParam_UsedImplementation=32 Bit Floating Point  x2c_cfg_enableStaticId=off  x2c_cfg_staticId=1  x2c_cfg_enableCot=off  BlockName=Constant
      settings: SourceProductName=X2C General
  Voltage Sensor : fl_lib/Electrical/Electrical Sensors/Voltage Sensor
  current : General/Gain  Gain=-1.0  M2CAutoParam_UsedImplementation=32 Bit Floating Point  x2c_cfg_enableStaticId=off  x2c_cfg_staticId=1  x2c_cfg_enableCot=off  BlockName=Gain
      settings: SourceProductName=X2C General
  torgue : Step  Time=2  After=1.0  SampleTime=0
  uGain : General/uGain  Gain=pp  M2CAutoParam_UsedImplementation=32 Bit Floating Point  x2c_cfg_enableStaticId=off  x2c_cfg_staticId=1  x2c_cfg_enableCot=off  BlockName=uGain
      settings: SourceProductName=X2C General
  uI : Control/uI  Ki=1  ts_fact=1.0  M2CAutoParam_UsedImplementation=32 Bit Floating Point  x2c_cfg_enableStaticId=off  x2c_cfg_staticId=1  x2c_cfg_enableCot=off  BlockName=uI
      settings: SourceProductName=X2C Control
  Out1 : Outport
  Out2 : Outport  Port=2
  tag scope: DutyABC=global, IndMotorMeasures=global, Ud=global
  wires:
  [DutyABC] -> Conv1/1
  [DutyABC_DC] -> Conv3/1
  PS-Simulink Converter6/1 -> [Ud]  "voltage"
  PS-Simulink Converter3/1 -> [VoltagesABC]  "voltage"
  PS-Simulink Converter4/1 -> [CurrentsABC]  "current"
  PS-Simulink Converter8/1 -> [CurrentsABC_DC]  "current"
  PS-Simulink Converter7/1 -> Goto2/1  "voltage"
  PS-Simulink Converter1/1 -> Display1/1  "reactive power"
  PS-Simulink Converter9/1 -> Display3/1  "active power"
  PS-Simulink Converter2/1 -> [IndMotorMeasures]
  Constant/1 -> Conv2/1
  Constant6/1 -> Simulink-PS Converter1/1
  PS-Simulink Converter5/1 -> [W], Gain/1  "w"
  Gain/1 -> Scope1/1, Display/1
  PS-Simulink Converter10/1 -> Scope9/2, Interpreted MATLAB Function/1, Scope1/2  "a"
  [Ud] -> Unit Delay1/1
  Unit Delay1/1 -> InVdc-2/1
  torgue/1 -> InTorque-2/1
  Demux2/1 -> InCurrentA-2/1
  Demux2/2 -> InCurrentB-2/1
  Demux2/3 -> InCurrentC-2/1
  Unit Delay2/1 -> Demux2/1
  [CurrentsABC_DC] -> Unit Delay2/1
  [W] -> InOme-2/1  "angular velecity"
  [A] -> InPhi-2/1  "angle"
  InTorque-2/1 -> 1/cfi/1
  1/cfi/1 -> current/1
  InCurrentA-2/1 -> Sub/2, Scope18/2
  current/1 -> Scope18/1, Sub/1
  Sub/1 -> Scope2/1, PI regulátor/1
  Constant4/1 -> PI regulátor/2
  Constant3/1 -> PI regulátor/3
  PI regulátor/1 -> Scope2/2, Div1/1
  Mux1/1 -> [DutyABC_DC]
  Div1/1 -> OutDutyA1/1, Negation/1, Scope10/2
  Constant1/1 -> OutDutyC1/1
  Negation/1 -> OutDutyB1/1
  OutDutyA1/1 -> Mux1/1
  OutDutyB1/1 -> Mux1/2
  OutDutyC1/1 -> Mux1/3
  InVdc-2/1 -> Scope10/1, Saturation/1
  Saturation/1 -> Div1/2
  InCurrentB-2/1 -> Terminator4/1
  InCurrentC-2/1 -> Terminator1/1
  InOme-2/1 -> Terminator2/1
  InPhi-2/1 -> Terminator3/1
  Demux/2 -> InCurrentB/1
  [CurrentsABC] -> Demux/1
  Demux/1 -> InCurrentA/1
  Demux/3 -> InCurrentC/1
  [Ud] -> Unit Delay/1
  Unit Delay/1 -> InVdc/1
  [W] -> InPhi/1  "angular velecity"
  [A] -> InOme/1  "angle"
  InPhi/1 -> uGain/1
  InOme/1 -> Terminator8/1
  InCurrentA/1 -> [A1], ClarkeNPark/1
  InCurrentB/1 -> ClarkeNPark/2
  InCurrentC/1 -> ClarkeNPark/3, [C1]
  ClarkeNPark/1 -> Scope3/1
  ClarkeNPark/2 -> Scope3/2
  Voltage/1 -> Mult/1
  1/f/1 -> Mult/2
  Frequency/1 -> Gain2/1, 1/f/1
  Mult/1 -> Gain1/1
  Gain1/1 -> Div/1
  Div/1 -> Saturation2/1
  Saturation2/1 -> InvPark/1
  InvPark/1 -> Space Vector Modulation/1
  InvPark/2 -> Space Vector Modulation/2
  OutDutyA/1 -> Mux/1
  OutDutyC/1 -> Mux/3
  Mux/1 -> [DutyABC]
  OutDutyB/1 -> Mux/2
  Space Vector Modulation/1 -> [A2], OutDutyA/1
  Space Vector Modulation/2 -> OutDutyB/1, [B2]
  Space Vector Modulation/3 -> [C2], OutDutyC/1
  Amplitude1/1 -> InvPark/2
  Init/1 -> uI/2
  Gain2/1 -> uI/1
  Enable/1 -> uI/3
  uI/1 -> InvPark/3, Scope4/1, ClarkeNPark/4
  InVdc/1 -> Saturation1/1
  Saturation1/1 -> [ABC], Div/2
  Mult3/1 -> Add1/1
  Mult5/1 -> Add1/2
  uGain/1 -> Scope4/2
  [A1] -> Mult3/1
  [C1] -> Mult5/1
  Gain5/1 -> Mult2/2
  Gain4/1 -> Mult1/2
  Delay/1 -> Gain4/1
  Delay1/1 -> Gain5/1
  Sub1/1 -> Delay/1
  Sub2/1 -> Delay1/1
  [A2] -> Sub1/1
  [C2] -> Sub2/1
  [B2] -> Sub2/2, Sub1/2
  [ABC] -> Mult1/1, Mult2/1
  Mult1/1 -> Mult3/2
  Mult2/1 -> Mult5/2
  [VoltagesABC] -> Demux5/1
  [CurrentsABC] -> Demux6/1
  Demux5/2 -> Gain3/1
  Gain3/1 -> Product1/1
  Demux6/3 -> Product1/2
  Demux5/1 -> Product/1
  Demux6/1 -> Product/2
  Demux5/3 -> Terminator/1
  Demux6/2 -> Terminator5/1
  Product/1 -> Add/1
  Product1/1 -> Add/2
  Add/1 -> Display4/1, Scope15/2
  Add1/1 -> Scope15/1
  Interpreted MATLAB Function/1 -> Scope9/1, [A]
  [W] -> Product2/1
  PS-Simulink Converter11/1 -> Scope12/2, Product2/2  "T"
  Product2/1 -> Scope12/1
  Demux1/6 -> Scope7/1  "ids"
  [IndMotorMeasures] -> Demux1/1
  Demux1/1 -> Scope5/1  "torgue"
  Demux1/8 -> Out2/1  "i0s"
  Demux1/2 -> Scope5/2  "velocity"
  Demux1/7 -> Scope7/2  "iqs"
  Demux1/3 -> Scope6/1  "vds"
  Demux1/5 -> Out1/1  "v0s"
  Demux1/4 -> Scope6/2  "vqs"
  connections:
  Converter (Three-Phase)-1/RConn1 -- Solver Configuration/RConn1 -- DC Voltage Source/LConn1 -- Voltage Sensor/LConn1 -- Converter (Three-Phase)-2/RConn1
  Converter (Three-Phase)-1/RConn2 -- GND/LConn1 -- Voltage Sensor/RConn2 -- DC Voltage Source/RConn1 -- Converter (Three-Phase)-2/RConn2
  AV Sensor (Three-Phase)-1/LConn1 -- Converter (Three-Phase)-1/LConn2
  Conv1/RConn1 -- Converter (Three-Phase)-1/LConn1
  Conv3/RConn1 -- Converter (Three-Phase)-2/LConn1
  AV Sensor (Three-Phase)-2/LConn1 -- Converter (Three-Phase)-2/LConn2
  PS-Simulink Converter6/LConn1 -- Voltage Sensor/RConn1
  PS-Simulink Converter3/LConn1 -- AV Sensor (Three-Phase)-1/RConn1
  PS-Simulink Converter4/LConn1 -- AV Sensor (Three-Phase)-1/RConn2
  PS-Simulink Converter7/LConn1 -- AV Sensor (Three-Phase)-2/RConn1
  PS-Simulink Converter8/LConn1 -- AV Sensor (Three-Phase)-2/RConn2
  Power Sensor (Three-Phase)/LConn1 -- AV Sensor (Three-Phase)-1/RConn3
  PS-Simulink Converter1/LConn1 -- Power Sensor (Three-Phase)/LConn3
  PS-Simulink Converter9/LConn1 -- Power Sensor (Three-Phase)/LConn2
  Induction Machine Squirrel Cage1/RConn2 -- Phase Permute/LConn1 -- Power Sensor (Three-Phase)/RConn1
  AV Sensor (Three-Phase)-2/RConn3 -- Phase Splitter/LConn1
  Phase Splitter/RConn3 -- Open Circuit/LConn1
  PS-Simulink Converter2/LConn1 -- Induction Machine Squirrel Cage1/RConn1
  Floating Neutral (Three-Phase)/LConn1 -- SPDT Switch (Three-Phase)/RConn1
  Phase Permute/RConn1 -- SPDT Switch (Three-Phase)/RConn2
  SPDT Switch (Three-Phase)/LConn2 -- Induction Machine Squirrel Cage1/RConn3
  Conv2/RConn1 -- SPDT Switch (Three-Phase)/LConn1
  Induction Machine Squirrel Cage1/LConn1 -- Ideal Torque Sensor/LConn1 -- Ideal Torque Source/LConn1 -- Ideal Rotational Motion Sensor/LConn1 -- Inertia/LConn1
  Mechanical Rotational Reference/LConn1 -- Induction Machine Squirrel Cage1/LConn2
  DC Motor/LConn2 -- Ideal Torque Sensor/RConn1
  Mechanical Rotational Reference2/LConn1 -- Ideal Rotational Motion Sensor/RConn1
  Mechanical Rotational Reference1/LConn1 -- DC Motor/RConn2 -- Ideal Torque Source/RConn2
  Simulink-PS Converter1/RConn1 -- Ideal Torque Source/RConn1
  PS-Simulink Converter5/LConn1 -- Ideal Rotational Motion Sensor/RConn2
  PS-Simulink Converter10/LConn1 -- Ideal Rotational Motion Sensor/RConn3
  Phase Splitter/RConn1 -- DC Motor/LConn1
  Phase Splitter/RConn2 -- DC Motor/RConn1
  Ideal Torque Sensor/RConn2 -- PS-Simulink Converter11/LConn1
